simulink model "Position_Motor_Controller"  (R2018b)
settings: Solver=VariableStepAuto  StartTime=0.0  StopTime=10.0  RelTol=1e-3
values from neighbouring files (symbols this model uses):
  b = 22.5    [DC_Simulink.m]
  K = 0.055    [DC_Servomotor_Code.m]    (also in DC_Simulink.m = 0.109)
  L = 5.02E-3    (= 0.00502)    [DC_Servomotor_Code.m]    (also in DC_Simulink.m = 0.000625)
  R = 41.5    [DC_Servomotor_Code.m]    (also in DC_Simulink.m = 0.522)
  Tload = TL(1,i)    [DC_Simulink.m]
undefined symbols (not defined in the file or in its folder): Jm
libraries: simulink x7
settings Model: Creator=james.quan.166  LastModifiedBy=James

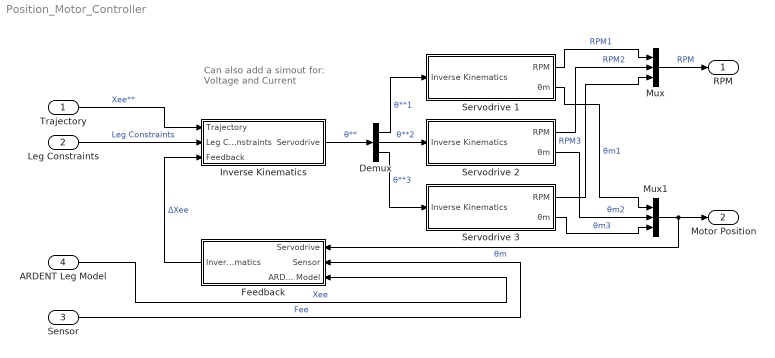
== system Position_Motor_Controller ==
  note: Can also add a simout for:
      | Voltage and Current
  Trajectory : Inport
  Leg Constraints : Inport  Port=2
  Sensor : Inport  Port=3
  ARDENT Leg Model : Inport  Port=4
  Demux : Demux  Outputs=3
  Feedback : Subsystem
  Inverse Kinematics : Subsystem
  Mux : Mux  Inputs=3
  Mux1 : Mux  Inputs=3
  Servodrive 1 : Subsystem
  Servodrive 2 : Subsystem
  Servodrive 3 : Subsystem
  RPM : Outport
  Motor Position : Outport  Port=2
  wires:
  Leg Constraints/1 -> Inverse Kinematics/2(Leg Constraints)  "Leg Constraints"
  Mux/1 -> RPM/1  "RPM"
  Feedback/1(Inverse Kinematics) -> Inverse Kinematics/3(Feedback)  "ΔXee"
  Mux1/1 -> Feedback/1(Servodrive), Motor Position/1  "θm"
  Sensor/1 -> Feedback/2(Sensor)  "Fee"
  Trajectory/1 -> Inverse Kinematics/1(Trajectory)  "Xee**"
  Inverse Kinematics/1(Servodrive) -> Demux/1  "θ**"
  ARDENT Leg Model/1 -> Feedback/3(ARDENT Leg Model)  "Xee"
  Servodrive 2/1(RPM) -> Mux/2  "RPM2"
  Demux/2 -> Servodrive 2/1(Inverse Kinematics)  "θ**2"
  Demux/1 -> Servodrive 1/1(Inverse Kinematics)  "θ**1"
  Demux/3 -> Servodrive 3/1(Inverse Kinematics)  "θ**3"
  Servodrive 3/1(RPM) -> Mux/3  "RPM3"
  Servodrive 3/2(θm) -> Mux1/3  "θm3"
  Servodrive 1/1(RPM) -> Mux/1  "RPM1"
  Servodrive 2/2(θm) -> Mux1/2  "θm2"
  Servodrive 1/2(θm) -> Mux1/1  "θm1"

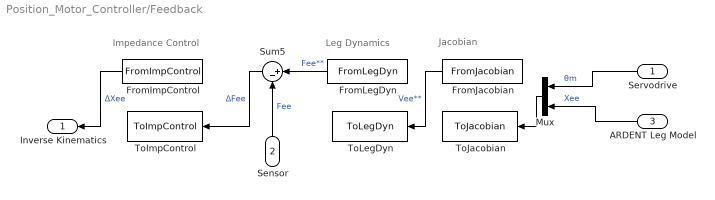
== system Position_Motor_Controller/Feedback ==
  note: Impedance Control
  note: Leg Dynamics
  note: Jacobian
  Servodrive : Inport
  Sensor : Inport  Port=2
  ARDENT Leg Model : Inport  Port=3
  FromImpControl : FromWorkspace  VariableName=FromImpControl  SampleTime=0
  FromJacobian : FromWorkspace  VariableName=FromJacobian  SampleTime=0
  FromLegDyn : FromWorkspace  VariableName=FromLegDyn  SampleTime=0
  Mux : Mux  Inputs=2
  Sum5 : Sum  Inputs=|+-
  ToImpControl : ToWorkspace  VariableName=ToImpControl  SaveFormat=Timeseries  SampleTime=-1
  ToJacobian : ToWorkspace  VariableName=ToJacobian  SaveFormat=Timeseries  SampleTime=-1
  ToLegDyn : ToWorkspace  VariableName=ToLegDyn  SaveFormat=Timeseries  SampleTime=-1
  Inverse Kinematics : Outport
  wires:
  Sensor/1 -> Sum5/2  "Fee"
  ARDENT Leg Model/1 -> Mux/2  "Xee"
  Servodrive/1 -> Mux/1  "θm"
  Mux/1 -> ToJacobian/1
  FromLegDyn/1 -> Sum5/1  "Fee**"
  FromJacobian/1 -> ToLegDyn/1  "Vee**"
  Sum5/1 -> ToImpControl/1  "ΔFee"
  FromImpControl/1 -> Inverse Kinematics/1  "ΔXee"

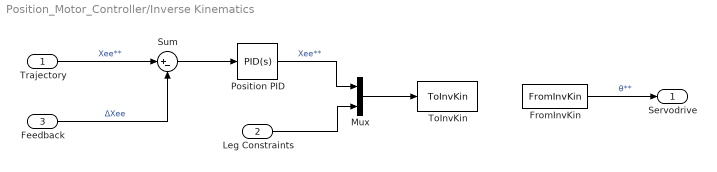
== system Position_Motor_Controller/Inverse Kinematics ==
  Trajectory : Inport
  Leg Constraints : Inport  Port=2
  Feedback : Inport  Port=3
  FromInvKin : FromWorkspace  VariableName=FromInvKin  SampleTime=0
  Mux : Mux  Inputs=2
  Position PID : simulink/Continuous/PID Controller  Controller=PID  Form=Parallel  TimeDomain=Continuous-time  SampleTime=-1  IntegratorMethod=Forward Euler  FilterMethod=Forward Euler  ControllerParametersSource=internal  P=1  I=1  D=0  UseFilter=on  N=100  TunerSelectOption=Transfer Function Based (PID Tuner App)  InitialConditionSource=internal  InitialConditionForIntegrator=0  InitialConditionForFilter=0  DifferentiatorICPrevScaledInput=0  ExternalReset=none  TrackingMode=off  Kt=1  LimitOutput=off  UpperSaturationLimit=inf  LowerSaturationLimit=-inf  LinearizeAsGain=on  AntiWindupMode=none  Kb=1  POutMin=[]  POutMax=[]  IOutMin=[]  IOutMax=[]  DOutMin=[]  DOutMax=[]  NOutMin=[]  NOutMax=[]  SumOutMin=[]  SumOutMax=[]  SaturationOutMin=[]  SaturationOutMax=[]  PParamMin=[]  PParamMax=[]  IParamMin=[]  IParamMax=[]  DParamMin=[]  DParamMax=[]  NParamMin=[]  NParamMax=[]  KbParamMin=[]  KbParamMax=[]  KtParamMin=[]  KtParamMax=[]  KbOutMin=[]  KbOutMax=[]  KtOutMin=[]  KtOutMax=[]  IntegratorOutMin=[]  IntegratorOutMax=[]  FilterOutMin=[]  FilterOutMax=[]  SumI1OutMin=[]  SumI1OutMax=[]  SumI2OutMin=[]  SumI2OutMax=[]  SumI3OutMin=[]  SumI3OutMax=[]  SumI4OutMin=[]  SumI4OutMax=[]  SumDOutMin=[]  SumDOutMax=[]  DifferentiatorOutMin=[]  DifferentiatorOutMax=[]  FilterDiffOutCoefMin=[]  FilterDiffOutCoefMax=[]  ReciprocalOutMin=[]  ReciprocalOutMax=[]  SumDenOutMin=[]  SumDenOutMax=[]  SumNumOutMin=[]  SumNumOutMax=[]  DivideOutMin=[]  DivideOutMax=[]  IntegratorContinuousStateAttributes=''  IntegratorStateMustResolveToSignalObject=off  IntegratorRTWStateStorageClass=Auto  FilterContinuousStateAttributes=''  FilterStateMustResolveToSignalObject=off  FilterRTWStateStorageClass=Auto  ParallelPVariant=InternalParameters  IdealPVariant=Disabled  IVariant=InternalParameters  DVariant=InternalParameters  IntegratorVariant=Continuous  SatVariant=Disabled  AWVariant=Passthrough  PCopyVariant=Disabled  TRVariant=Disabled  FdbkBlocksVariant=Forward  IdealPFdbkVariant=Disabled  SatFdbkVariant=Disabled  DerivativeFilterVariant=ContFilter  NVariant=InternalParameters  NCopyVariant=Disabled  FilterICVariant=InternalICsFilter  IntegratorICVariant=InternalICs  ExternalResetVariant=Disabled  TRSumVariant=Passthrough  SumFdbkVariant=Disabled  SumVariant=Sum_PID
  Sum : Sum  Inputs=|+-
  ToInvKin : ToWorkspace  VariableName=ToInvKin  SaveFormat=Timeseries  SampleTime=-1
  Servodrive : Outport
  wires:
  Trajectory/1 -> Sum/1  "Xee**"
  Leg Constraints/1 -> Mux/2
  Feedback/1 -> Sum/2  "ΔXee"
  Mux/1 -> ToInvKin/1
  FromInvKin/1 -> Servodrive/1  "θ**"
  Sum/1 -> Position PID/1
  Position PID/1 -> Mux/1  "Xee**"

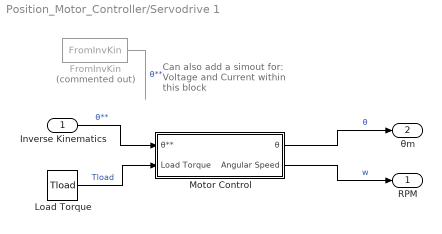
== system Position_Motor_Controller/Servodrive 1 ==
  note: Can also add a simout for:
      | Voltage and Current
      | within this block
  Inverse Kinematics : Inport
  FromInvKin : FromWorkspace  Commented=on  VariableName=FromInvKin  SampleTime=0
  Load Torque : Constant  Value=Tload
  Motor Control : Subsystem
  RPM : Outport
  θm : Outport  Port=2
  wires:
  Inverse Kinematics/1 -> Motor Control/1(θ**)  "θ**"
  FromInvKin/1 -> ?  "θ**"
  Load Torque/1 -> Motor Control/2(Load Torque)  "Tload"
  Motor Control/1(θ) -> θm/1  "θ"
  Motor Control/2(Angular Speed) -> RPM/1  "w"

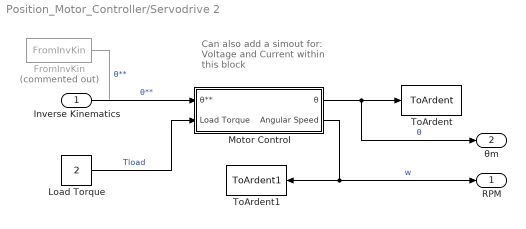
== system Position_Motor_Controller/Servodrive 2 ==
  note: Can also add a simout for:
      | Voltage and Current
      | within this block
  Inverse Kinematics : Inport
  FromInvKin : FromWorkspace  Commented=on  VariableName=FromInvKin  SampleTime=0
  Load Torque : Constant  Value=2
  Motor Control : Subsystem
  ToArdent : ToWorkspace  VariableName=ToArdent  SaveFormat=Timeseries  SampleTime=-1
  ToArdent1 : ToWorkspace  VariableName=ToArdent1  SaveFormat=Timeseries  SampleTime=-1
  RPM : Outport
  θm : Outport  Port=2
  wires:
  Inverse Kinematics/1 -> Motor Control/1(θ**)  "θ**"
  FromInvKin/1 -> ?  "θ**"
  Load Torque/1 -> Motor Control/2(Load Torque)  "Tload"
  Motor Control/1(θ) -> θm/1, ToArdent/1  "θ"
  Motor Control/2(Angular Speed) -> ToArdent1/1, RPM/1  "w"

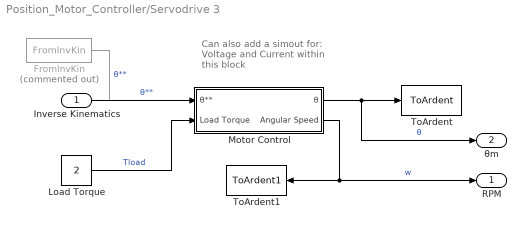
== system Position_Motor_Controller/Servodrive 3 ==
  note: Can also add a simout for:
      | Voltage and Current
      | within this block
  Inverse Kinematics : Inport
  FromInvKin : FromWorkspace  Commented=on  VariableName=FromInvKin  SampleTime=0
  Load Torque : Constant  Value=2
  Motor Control : Subsystem
  ToArdent : ToWorkspace  VariableName=ToArdent  SaveFormat=Timeseries  SampleTime=-1
  ToArdent1 : ToWorkspace  VariableName=ToArdent1  SaveFormat=Timeseries  SampleTime=-1
  RPM : Outport
  θm : Outport  Port=2
  wires:
  Inverse Kinematics/1 -> Motor Control/1(θ**)  "θ**"
  FromInvKin/1 -> ?  "θ**"
  Load Torque/1 -> Motor Control/2(Load Torque)  "Tload"
  Motor Control/1(θ) -> θm/1, ToArdent/1  "θ"
  Motor Control/2(Angular Speed) -> ToArdent1/1, RPM/1  "w"

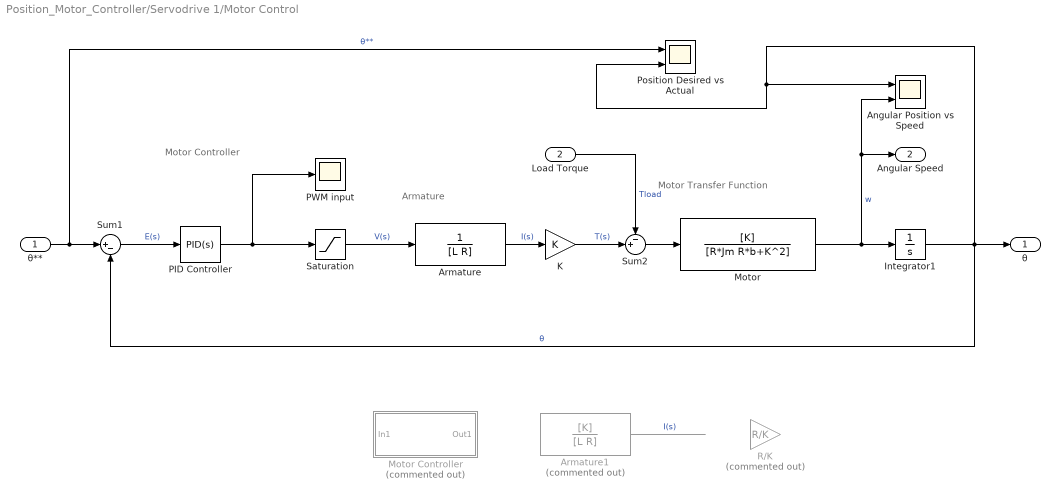
== system Position_Motor_Controller/Servodrive 1/Motor Control ==
  note: Armature
  note: Motor Transfer Function
  note: Motor Controller
  θ** : Inport
  Load Torque : Inport  Port=2
  Angular Position vs Speed : Scope  NumInputPorts=2
  Armature : TransferFcn  Denominator=[L R]
  Armature1 : TransferFcn  Commented=on  Numerator=[K]  Denominator=[L R]
  Integrator1 : Integrator
  K : Gain  Gain=K
  Motor : TransferFcn  Numerator=[K]  Denominator=[R*Jm R*b+K^2]
  Motor Controller : Subsystem  Commented=on
  PID Controller : simulink/Continuous/PID Controller  Controller=PID  Form=Parallel  TimeDomain=Continuous-time  SampleTime=-1  IntegratorMethod=Forward Euler  FilterMethod=Forward Euler  ControllerParametersSource=internal  P=965  I=2000  D=0  UseFilter=on  N=1330  TunerSelectOption=Transfer Function Based (PID Tuner App)  InitialConditionSource=internal  InitialConditionForIntegrator=0  InitialConditionForFilter=0  DifferentiatorICPrevScaledInput=0  ExternalReset=none  TrackingMode=off  Kt=1  LimitOutput=off  UpperSaturationLimit=inf  LowerSaturationLimit=-inf  LinearizeAsGain=on  AntiWindupMode=none  Kb=1  POutMin=[]  POutMax=[]  IOutMin=[]  IOutMax=[]  DOutMin=[]  DOutMax=[]  NOutMin=[]  NOutMax=[]  SumOutMin=[]  SumOutMax=[]  SaturationOutMin=[]  SaturationOutMax=[]  PParamMin=[]  PParamMax=[]  IParamMin=[]  IParamMax=[]  DParamMin=[]  DParamMax=[]  NParamMin=[]  NParamMax=[]  KbParamMin=[]  KbParamMax=[]  KtParamMin=[]  KtParamMax=[]  KbOutMin=[]  KbOutMax=[]  KtOutMin=[]  KtOutMax=[]  IntegratorOutMin=[]  IntegratorOutMax=[]  FilterOutMin=[]  FilterOutMax=[]  SumI1OutMin=[]  SumI1OutMax=[]  SumI2OutMin=[]  SumI2OutMax=[]  SumI3OutMin=[]  SumI3OutMax=[]  SumI4OutMin=[]  SumI4OutMax=[]  SumDOutMin=[]  SumDOutMax=[]  DifferentiatorOutMin=[]  DifferentiatorOutMax=[]  FilterDiffOutCoefMin=[]  FilterDiffOutCoefMax=[]  ReciprocalOutMin=[]  ReciprocalOutMax=[]  SumDenOutMin=[]  SumDenOutMax=[]  SumNumOutMin=[]  SumNumOutMax=[]  DivideOutMin=[]  DivideOutMax=[]  IntegratorContinuousStateAttributes=''  IntegratorStateMustResolveToSignalObject=off  IntegratorRTWStateStorageClass=Auto  FilterContinuousStateAttributes=''  FilterStateMustResolveToSignalObject=off  FilterRTWStateStorageClass=Auto  ParallelPVariant=InternalParameters  IdealPVariant=Disabled  IVariant=InternalParameters  DVariant=InternalParameters  IntegratorVariant=Continuous  SatVariant=Disabled  AWVariant=Passthrough  PCopyVariant=Disabled  TRVariant=Disabled  FdbkBlocksVariant=Forward  IdealPFdbkVariant=Disabled  SatFdbkVariant=Disabled  DerivativeFilterVariant=ContFilter  NVariant=InternalParameters  NCopyVariant=Disabled  FilterICVariant=InternalICsFilter  IntegratorICVariant=InternalICs  ExternalResetVariant=Disabled  TRSumVariant=Passthrough  SumFdbkVariant=Disabled  SumVariant=Sum_PID
  PWM input : Scope
  Position Desired vs Actual : Scope  NumInputPorts=2
  "R/K " : Gain  Commented=on  Gain=R/K
  "Saturation " : Saturate  UpperLimit=127  LowerLimit=-127
  Sum1 : Sum  Inputs=|+-
  Sum2 : Sum  Inputs=-+|
  θ : Outport
  Angular Speed : Outport  Port=2
  wires:
  θ**/1 -> Position Desired vs Actual/1, Sum1/1  "θ**"
  Sum2/1 -> Motor/1
  Motor/1 -> Integrator1/1, Angular Speed/1, Angular Position vs Speed/2  "w"
  Integrator1/1 -> θ/1, Sum1/2, Position Desired vs Actual/2, Angular Position vs Speed/1  "θ"
  Load Torque/1 -> Sum2/1  "Tload"
  Sum1/1 -> PID Controller/1  "E(s)"
  "Saturation "/1 -> Armature/1  "V(s)"
  K/1 -> Sum2/2  "T(s)"
  Armature/1 -> K/1  "I(s)"
  PID Controller/1 -> "Saturation "/1, PWM input/1
  Armature1/1 -> ?  "I(s)"

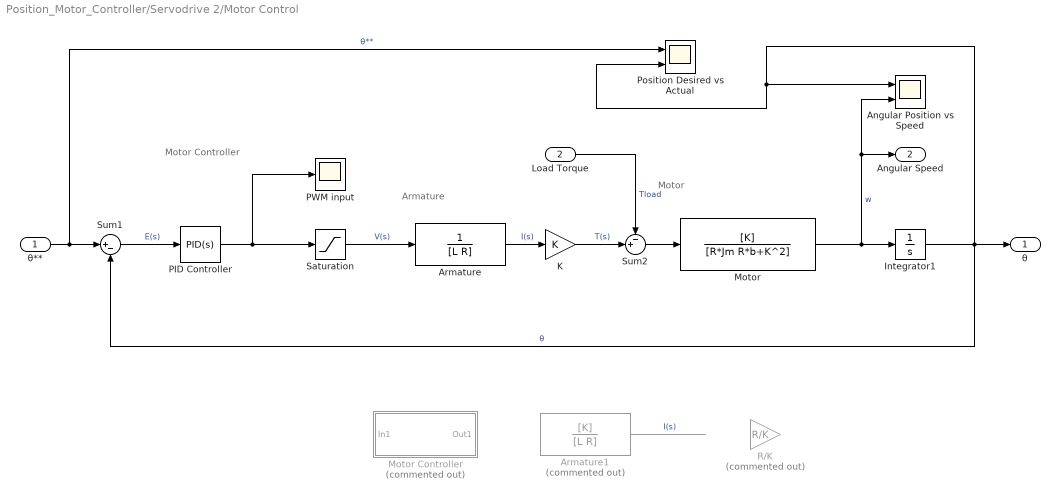
== system Position_Motor_Controller/Servodrive 2/Motor Control ==
  note: Armature
  note: Motor
  note: Motor Controller
  θ** : Inport
  Load Torque : Inport  Port=2
  Angular Position vs Speed : Scope  NumInputPorts=2
  Armature : TransferFcn  Denominator=[L R]
  Armature1 : TransferFcn  Commented=on  Numerator=[K]  Denominator=[L R]
  Integrator1 : Integrator
  K : Gain  Gain=K
  Motor : TransferFcn  Numerator=[K]  Denominator=[R*Jm R*b+K^2]
  Motor Controller : Subsystem  Commented=on
  PID Controller : simulink/Continuous/PID Controller  Controller=PID  Form=Parallel  TimeDomain=Continuous-time  SampleTime=-1  IntegratorMethod=Forward Euler  FilterMethod=Forward Euler  ControllerParametersSource=internal  P=965  I=2000  D=0  UseFilter=on  N=1330  TunerSelectOption=Transfer Function Based (PID Tuner App)  InitialConditionSource=internal  InitialConditionForIntegrator=0  InitialConditionForFilter=0  DifferentiatorICPrevScaledInput=0  ExternalReset=none  TrackingMode=off  Kt=1  LimitOutput=off  UpperSaturationLimit=inf  LowerSaturationLimit=-inf  LinearizeAsGain=on  AntiWindupMode=none  Kb=1  POutMin=[]  POutMax=[]  IOutMin=[]  IOutMax=[]  DOutMin=[]  DOutMax=[]  NOutMin=[]  NOutMax=[]  SumOutMin=[]  SumOutMax=[]  SaturationOutMin=[]  SaturationOutMax=[]  PParamMin=[]  PParamMax=[]  IParamMin=[]  IParamMax=[]  DParamMin=[]  DParamMax=[]  NParamMin=[]  NParamMax=[]  KbParamMin=[]  KbParamMax=[]  KtParamMin=[]  KtParamMax=[]  KbOutMin=[]  KbOutMax=[]  KtOutMin=[]  KtOutMax=[]  IntegratorOutMin=[]  IntegratorOutMax=[]  FilterOutMin=[]  FilterOutMax=[]  SumI1OutMin=[]  SumI1OutMax=[]  SumI2OutMin=[]  SumI2OutMax=[]  SumI3OutMin=[]  SumI3OutMax=[]  SumI4OutMin=[]  SumI4OutMax=[]  SumDOutMin=[]  SumDOutMax=[]  DifferentiatorOutMin=[]  DifferentiatorOutMax=[]  FilterDiffOutCoefMin=[]  FilterDiffOutCoefMax=[]  ReciprocalOutMin=[]  ReciprocalOutMax=[]  SumDenOutMin=[]  SumDenOutMax=[]  SumNumOutMin=[]  SumNumOutMax=[]  DivideOutMin=[]  DivideOutMax=[]  IntegratorContinuousStateAttributes=''  IntegratorStateMustResolveToSignalObject=off  IntegratorRTWStateStorageClass=Auto  FilterContinuousStateAttributes=''  FilterStateMustResolveToSignalObject=off  FilterRTWStateStorageClass=Auto  ParallelPVariant=InternalParameters  IdealPVariant=Disabled  IVariant=InternalParameters  DVariant=InternalParameters  IntegratorVariant=Continuous  SatVariant=Disabled  AWVariant=Passthrough  PCopyVariant=Disabled  TRVariant=Disabled  FdbkBlocksVariant=Forward  IdealPFdbkVariant=Disabled  SatFdbkVariant=Disabled  DerivativeFilterVariant=ContFilter  NVariant=InternalParameters  NCopyVariant=Disabled  FilterICVariant=InternalICsFilter  IntegratorICVariant=InternalICs  ExternalResetVariant=Disabled  TRSumVariant=Passthrough  SumFdbkVariant=Disabled  SumVariant=Sum_PID
  PWM input : Scope
  Position Desired vs Actual : Scope  NumInputPorts=2
  "R/K " : Gain  Commented=on  Gain=R/K
  Saturation : Saturate  UpperLimit=127  LowerLimit=-127
  Sum1 : Sum  Inputs=|+-
  Sum2 : Sum  Inputs=-+|
  θ : Outport
  Angular Speed : Outport  Port=2
  wires:
  θ**/1 -> Position Desired vs Actual/1, Sum1/1  "θ**"
  Sum2/1 -> Motor/1
  Motor/1 -> Integrator1/1, Angular Speed/1, Angular Position vs Speed/2  "w"
  Integrator1/1 -> θ/1, Sum1/2, Position Desired vs Actual/2, Angular Position vs Speed/1  "θ"
  Load Torque/1 -> Sum2/1  "Tload"
  Sum1/1 -> PID Controller/1  "E(s)"
  Saturation/1 -> Armature/1  "V(s)"
  K/1 -> Sum2/2  "T(s)"
  Armature/1 -> K/1  "I(s)"
  PID Controller/1 -> Saturation/1, PWM input/1
  Armature1/1 -> ?  "I(s)"

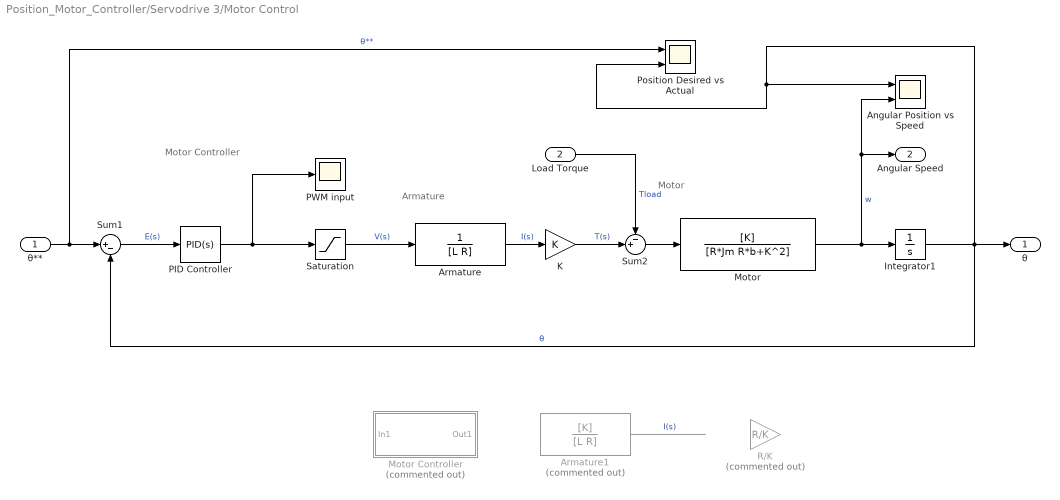
== system Position_Motor_Controller/Servodrive 3/Motor Control ==
  note: Armature
  note: Motor
  note: Motor Controller
  θ** : Inport
  Load Torque : Inport  Port=2
  Angular Position vs Speed : Scope  NumInputPorts=2
  Armature : TransferFcn  Denominator=[L R]
  Armature1 : TransferFcn  Commented=on  Numerator=[K]  Denominator=[L R]
  Integrator1 : Integrator
  K : Gain  Gain=K
  Motor : TransferFcn  Numerator=[K]  Denominator=[R*Jm R*b+K^2]
  Motor Controller : Subsystem  Commented=on
  PID Controller : simulink/Continuous/PID Controller  Controller=PID  Form=Parallel  TimeDomain=Continuous-time  SampleTime=-1  IntegratorMethod=Forward Euler  FilterMethod=Forward Euler  ControllerParametersSource=internal  P=965  I=2000  D=0  UseFilter=on  N=1330  TunerSelectOption=Transfer Function Based (PID Tuner App)  InitialConditionSource=internal  InitialConditionForIntegrator=0  InitialConditionForFilter=0  DifferentiatorICPrevScaledInput=0  ExternalReset=none  TrackingMode=off  Kt=1  LimitOutput=off  UpperSaturationLimit=inf  LowerSaturationLimit=-inf  LinearizeAsGain=on  AntiWindupMode=none  Kb=1  POutMin=[]  POutMax=[]  IOutMin=[]  IOutMax=[]  DOutMin=[]  DOutMax=[]  NOutMin=[]  NOutMax=[]  SumOutMin=[]  SumOutMax=[]  SaturationOutMin=[]  SaturationOutMax=[]  PParamMin=[]  PParamMax=[]  IParamMin=[]  IParamMax=[]  DParamMin=[]  DParamMax=[]  NParamMin=[]  NParamMax=[]  KbParamMin=[]  KbParamMax=[]  KtParamMin=[]  KtParamMax=[]  KbOutMin=[]  KbOutMax=[]  KtOutMin=[]  KtOutMax=[]  IntegratorOutMin=[]  IntegratorOutMax=[]  FilterOutMin=[]  FilterOutMax=[]  SumI1OutMin=[]  SumI1OutMax=[]  SumI2OutMin=[]  SumI2OutMax=[]  SumI3OutMin=[]  SumI3OutMax=[]  SumI4OutMin=[]  SumI4OutMax=[]  SumDOutMin=[]  SumDOutMax=[]  DifferentiatorOutMin=[]  DifferentiatorOutMax=[]  FilterDiffOutCoefMin=[]  FilterDiffOutCoefMax=[]  ReciprocalOutMin=[]  ReciprocalOutMax=[]  SumDenOutMin=[]  SumDenOutMax=[]  SumNumOutMin=[]  SumNumOutMax=[]  DivideOutMin=[]  DivideOutMax=[]  IntegratorContinuousStateAttributes=''  IntegratorStateMustResolveToSignalObject=off  IntegratorRTWStateStorageClass=Auto  FilterContinuousStateAttributes=''  FilterStateMustResolveToSignalObject=off  FilterRTWStateStorageClass=Auto  ParallelPVariant=InternalParameters  IdealPVariant=Disabled  IVariant=InternalParameters  DVariant=InternalParameters  IntegratorVariant=Continuous  SatVariant=Disabled  AWVariant=Passthrough  PCopyVariant=Disabled  TRVariant=Disabled  FdbkBlocksVariant=Forward  IdealPFdbkVariant=Disabled  SatFdbkVariant=Disabled  DerivativeFilterVariant=ContFilter  NVariant=InternalParameters  NCopyVariant=Disabled  FilterICVariant=InternalICsFilter  IntegratorICVariant=InternalICs  ExternalResetVariant=Disabled  TRSumVariant=Passthrough  SumFdbkVariant=Disabled  SumVariant=Sum_PID
  PWM input : Scope
  Position Desired vs Actual : Scope  NumInputPorts=2
  "R/K " : Gain  Commented=on  Gain=R/K
  Saturation : Saturate  UpperLimit=127  LowerLimit=-127
  Sum1 : Sum  Inputs=|+-
  Sum2 : Sum  Inputs=-+|
  θ : Outport
  Angular Speed : Outport  Port=2
  wires:
  θ**/1 -> Position Desired vs Actual/1, Sum1/1  "θ**"
  Sum2/1 -> Motor/1
  Motor/1 -> Integrator1/1, Angular Speed/1, Angular Position vs Speed/2  "w"
  Integrator1/1 -> θ/1, Sum1/2, Position Desired vs Actual/2, Angular Position vs Speed/1  "θ"
  Load Torque/1 -> Sum2/1  "Tload"
  Sum1/1 -> PID Controller/1  "E(s)"
  Saturation/1 -> Armature/1  "V(s)"
  K/1 -> Sum2/2  "T(s)"
  Armature/1 -> K/1  "I(s)"
  PID Controller/1 -> Saturation/1, PWM input/1
  Armature1/1 -> ?  "I(s)"

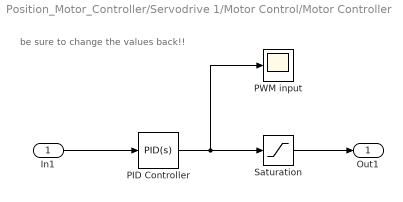
== system Position_Motor_Controller/Servodrive 1/Motor Control/Motor Controller ==
  note: be sure to change the values back!!
  In1 : Inport
  PID Controller : simulink/Continuous/PID Controller  Controller=PID  Form=Parallel  TimeDomain=Continuous-time  SampleTime=-1  IntegratorMethod=Forward Euler  FilterMethod=Forward Euler  ControllerParametersSource=internal  P=900  I=2000  D=10  UseFilter=on  N=1330  TunerSelectOption=Transfer Function Based (PID Tuner App)  InitialConditionSource=internal  InitialConditionForIntegrator=0  InitialConditionForFilter=0  DifferentiatorICPrevScaledInput=0  ExternalReset=none  TrackingMode=off  Kt=1  LimitOutput=off  UpperSaturationLimit=inf  LowerSaturationLimit=-inf  LinearizeAsGain=on  AntiWindupMode=none  Kb=1  POutMin=[]  POutMax=[]  IOutMin=[]  IOutMax=[]  DOutMin=[]  DOutMax=[]  NOutMin=[]  NOutMax=[]  SumOutMin=[]  SumOutMax=[]  SaturationOutMin=[]  SaturationOutMax=[]  PParamMin=[]  PParamMax=[]  IParamMin=[]  IParamMax=[]  DParamMin=[]  DParamMax=[]  NParamMin=[]  NParamMax=[]  KbParamMin=[]  KbParamMax=[]  KtParamMin=[]  KtParamMax=[]  KbOutMin=[]  KbOutMax=[]  KtOutMin=[]  KtOutMax=[]  IntegratorOutMin=[]  IntegratorOutMax=[]  FilterOutMin=[]  FilterOutMax=[]  SumI1OutMin=[]  SumI1OutMax=[]  SumI2OutMin=[]  SumI2OutMax=[]  SumI3OutMin=[]  SumI3OutMax=[]  SumI4OutMin=[]  SumI4OutMax=[]  SumDOutMin=[]  SumDOutMax=[]  DifferentiatorOutMin=[]  DifferentiatorOutMax=[]  FilterDiffOutCoefMin=[]  FilterDiffOutCoefMax=[]  ReciprocalOutMin=[]  ReciprocalOutMax=[]  SumDenOutMin=[]  SumDenOutMax=[]  SumNumOutMin=[]  SumNumOutMax=[]  DivideOutMin=[]  DivideOutMax=[]  IntegratorContinuousStateAttributes=''  IntegratorStateMustResolveToSignalObject=off  IntegratorRTWStateStorageClass=Auto  FilterContinuousStateAttributes=''  FilterStateMustResolveToSignalObject=off  FilterRTWStateStorageClass=Auto  ParallelPVariant=InternalParameters  IdealPVariant=Disabled  IVariant=InternalParameters  DVariant=InternalParameters  IntegratorVariant=Continuous  SatVariant=Disabled  AWVariant=Passthrough  PCopyVariant=Disabled  TRVariant=Disabled  FdbkBlocksVariant=Forward  IdealPFdbkVariant=Disabled  SatFdbkVariant=Disabled  DerivativeFilterVariant=ContFilter  NVariant=InternalParameters  NCopyVariant=Disabled  FilterICVariant=InternalICsFilter  IntegratorICVariant=InternalICs  ExternalResetVariant=Disabled  TRSumVariant=Passthrough  SumFdbkVariant=Disabled  SumVariant=Sum_PID
  PWM input : Scope
  Saturation : Saturate  UpperLimit=127  LowerLimit=-127
  Out1 : Outport
  wires:
  In1/1 -> PID Controller/1
  Saturation/1 -> Out1/1
  PID Controller/1 -> Saturation/1, PWM input/1

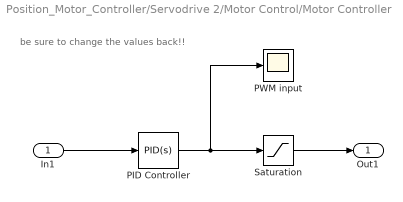
== system Position_Motor_Controller/Servodrive 2/Motor Control/Motor Controller ==
  note: be sure to change the values back!!
  In1 : Inport
  PID Controller : simulink/Continuous/PID Controller  Controller=PID  Form=Parallel  TimeDomain=Continuous-time  SampleTime=-1  IntegratorMethod=Forward Euler  FilterMethod=Forward Euler  ControllerParametersSource=internal  P=900  I=2000  D=10  UseFilter=on  N=1330  TunerSelectOption=Transfer Function Based (PID Tuner App)  InitialConditionSource=internal  InitialConditionForIntegrator=0  InitialConditionForFilter=0  DifferentiatorICPrevScaledInput=0  ExternalReset=none  TrackingMode=off  Kt=1  LimitOutput=off  UpperSaturationLimit=inf  LowerSaturationLimit=-inf  LinearizeAsGain=on  AntiWindupMode=none  Kb=1  POutMin=[]  POutMax=[]  IOutMin=[]  IOutMax=[]  DOutMin=[]  DOutMax=[]  NOutMin=[]  NOutMax=[]  SumOutMin=[]  SumOutMax=[]  SaturationOutMin=[]  SaturationOutMax=[]  PParamMin=[]  PParamMax=[]  IParamMin=[]  IParamMax=[]  DParamMin=[]  DParamMax=[]  NParamMin=[]  NParamMax=[]  KbParamMin=[]  KbParamMax=[]  KtParamMin=[]  KtParamMax=[]  KbOutMin=[]  KbOutMax=[]  KtOutMin=[]  KtOutMax=[]  IntegratorOutMin=[]  IntegratorOutMax=[]  FilterOutMin=[]  FilterOutMax=[]  SumI1OutMin=[]  SumI1OutMax=[]  SumI2OutMin=[]  SumI2OutMax=[]  SumI3OutMin=[]  SumI3OutMax=[]  SumI4OutMin=[]  SumI4OutMax=[]  SumDOutMin=[]  SumDOutMax=[]  DifferentiatorOutMin=[]  DifferentiatorOutMax=[]  FilterDiffOutCoefMin=[]  FilterDiffOutCoefMax=[]  ReciprocalOutMin=[]  ReciprocalOutMax=[]  SumDenOutMin=[]  SumDenOutMax=[]  SumNumOutMin=[]  SumNumOutMax=[]  DivideOutMin=[]  DivideOutMax=[]  IntegratorContinuousStateAttributes=''  IntegratorStateMustResolveToSignalObject=off  IntegratorRTWStateStorageClass=Auto  FilterContinuousStateAttributes=''  FilterStateMustResolveToSignalObject=off  FilterRTWStateStorageClass=Auto  ParallelPVariant=InternalParameters  IdealPVariant=Disabled  IVariant=InternalParameters  DVariant=InternalParameters  IntegratorVariant=Continuous  SatVariant=Disabled  AWVariant=Passthrough  PCopyVariant=Disabled  TRVariant=Disabled  FdbkBlocksVariant=Forward  IdealPFdbkVariant=Disabled  SatFdbkVariant=Disabled  DerivativeFilterVariant=ContFilter  NVariant=InternalParameters  NCopyVariant=Disabled  FilterICVariant=InternalICsFilter  IntegratorICVariant=InternalICs  ExternalResetVariant=Disabled  TRSumVariant=Passthrough  SumFdbkVariant=Disabled  SumVariant=Sum_PID
  PWM input : Scope
  Saturation : Saturate  UpperLimit=127  LowerLimit=-127
  Out1 : Outport
  wires:
  In1/1 -> PID Controller/1
  Saturation/1 -> Out1/1
  PID Controller/1 -> Saturation/1, PWM input/1

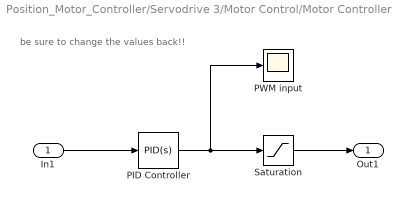
== system Position_Motor_Controller/Servodrive 3/Motor Control/Motor Controller ==
  note: be sure to change the values back!!
  In1 : Inport
  PID Controller : simulink/Continuous/PID Controller  Controller=PID  Form=Parallel  TimeDomain=Continuous-time  SampleTime=-1  IntegratorMethod=Forward Euler  FilterMethod=Forward Euler  ControllerParametersSource=internal  P=900  I=2000  D=10  UseFilter=on  N=1330  TunerSelectOption=Transfer Function Based (PID Tuner App)  InitialConditionSource=internal  InitialConditionForIntegrator=0  InitialConditionForFilter=0  DifferentiatorICPrevScaledInput=0  ExternalReset=none  TrackingMode=off  Kt=1  LimitOutput=off  UpperSaturationLimit=inf  LowerSaturationLimit=-inf  LinearizeAsGain=on  AntiWindupMode=none  Kb=1  POutMin=[]  POutMax=[]  IOutMin=[]  IOutMax=[]  DOutMin=[]  DOutMax=[]  NOutMin=[]  NOutMax=[]  SumOutMin=[]  SumOutMax=[]  SaturationOutMin=[]  SaturationOutMax=[]  PParamMin=[]  PParamMax=[]  IParamMin=[]  IParamMax=[]  DParamMin=[]  DParamMax=[]  NParamMin=[]  NParamMax=[]  KbParamMin=[]  KbParamMax=[]  KtParamMin=[]  KtParamMax=[]  KbOutMin=[]  KbOutMax=[]  KtOutMin=[]  KtOutMax=[]  IntegratorOutMin=[]  IntegratorOutMax=[]  FilterOutMin=[]  FilterOutMax=[]  SumI1OutMin=[]  SumI1OutMax=[]  SumI2OutMin=[]  SumI2OutMax=[]  SumI3OutMin=[]  SumI3OutMax=[]  SumI4OutMin=[]  SumI4OutMax=[]  SumDOutMin=[]  SumDOutMax=[]  DifferentiatorOutMin=[]  DifferentiatorOutMax=[]  FilterDiffOutCoefMin=[]  FilterDiffOutCoefMax=[]  ReciprocalOutMin=[]  ReciprocalOutMax=[]  SumDenOutMin=[]  SumDenOutMax=[]  SumNumOutMin=[]  SumNumOutMax=[]  DivideOutMin=[]  DivideOutMax=[]  IntegratorContinuousStateAttributes=''  IntegratorStateMustResolveToSignalObject=off  IntegratorRTWStateStorageClass=Auto  FilterContinuousStateAttributes=''  FilterStateMustResolveToSignalObject=off  FilterRTWStateStorageClass=Auto  ParallelPVariant=InternalParameters  IdealPVariant=Disabled  IVariant=InternalParameters  DVariant=InternalParameters  IntegratorVariant=Continuous  SatVariant=Disabled  AWVariant=Passthrough  PCopyVariant=Disabled  TRVariant=Disabled  FdbkBlocksVariant=Forward  IdealPFdbkVariant=Disabled  SatFdbkVariant=Disabled  DerivativeFilterVariant=ContFilter  NVariant=InternalParameters  NCopyVariant=Disabled  FilterICVariant=InternalICsFilter  IntegratorICVariant=InternalICs  ExternalResetVariant=Disabled  TRSumVariant=Passthrough  SumFdbkVariant=Disabled  SumVariant=Sum_PID
  PWM input : Scope
  Saturation : Saturate  UpperLimit=127  LowerLimit=-127
  Out1 : Outport
  wires:
  In1/1 -> PID Controller/1
  Saturation/1 -> Out1/1
  PID Controller/1 -> Saturation/1, PWM input/1
